simulink model "funkcija"  (R2015a)
settings: Solver=ode45  StartTime=0.0  StopTime=100.0  RelTol=1e-3
values from neighbouring files (symbols this model uses):
  teta1 = 0.5    [Parametri.m]
  teta2 = -0    (= 0)    [Parametri.m]
  v1 = 0    [Parametri.m]
  v2 = 0    [Parametri.m]
undefined symbols (not defined in the file or in its folder): A1, A2, A3, A4, l1, l2
settings Model: Creator=BLAGI  LastModifiedBy=BLAGI

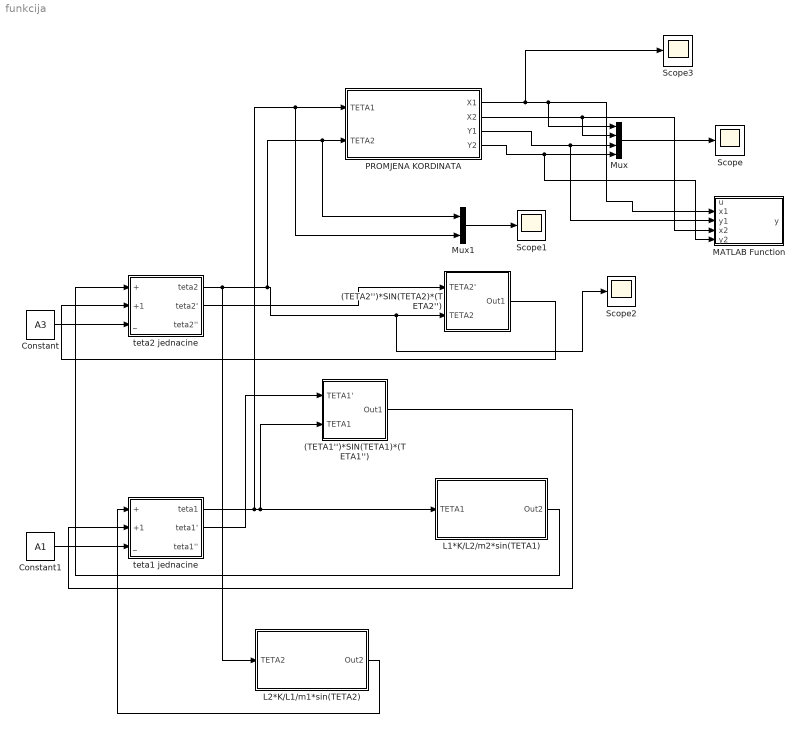
== system funkcija ==
  (TETA1'')*SIN(TETA1)*(TETA1'') : Subsystem
  (TETA2'')*SIN(TETA2)*(TETA2'') : Subsystem
  Constant : Constant  Value=A3
  Constant1 : Constant  Value=A1
  L1*K/L2/m2*sin(TETA1) : Subsystem
  L2*K/L1/m1*sin(TETA2) : Subsystem
  MATLAB Function : MATLAB Function  TreatAsAtomicUnit=on
  Mux : Mux
  Mux1 : Mux  Inputs=2
  "PROMJENA KORDINATA " : Subsystem
  Scope{,1..3} (4 alike) : Scope
      Scope settings: YMin=0  YMax=1
      Scope1 settings: YMin=0  YMax=1
      Scope2 settings: YMin=0  YMax=1  SaveName=ScopeData2
      Scope3 settings: YMin=0  YMax=1  SaveName=ScopeData3
  teta1 jednacine : Subsystem
  teta2 jednacine : Subsystem
  wires:
  Constant/1 -> teta2 jednacine/3(_)
  Constant1/1 -> teta1 jednacine/3(_)
  teta2 jednacine/1(teta2) -> L2*K/L1/m1*sin(TETA2)/1(TETA2), Mux1/1, "PROMJENA KORDINATA "/2(TETA2), Scope2/1, (TETA2'')*SIN(TETA2)*(TETA2'')/2(TETA2)
  (TETA2'')*SIN(TETA2)*(TETA2'')/1(Out1) -> teta2 jednacine/2(+1)
  L1*K/L2/m2*sin(TETA1)/1(Out2) -> teta2 jednacine/1(+)
  teta1 jednacine/2(teta1') -> (TETA1'')*SIN(TETA1)*(TETA1'')/1(TETA1')
  (TETA1'')*SIN(TETA1)*(TETA1'')/1(Out1) -> teta1 jednacine/2(+1)
  teta2 jednacine/2(teta2') -> (TETA2'')*SIN(TETA2)*(TETA2'')/1(TETA2')
  L2*K/L1/m1*sin(TETA2)/1(Out2) -> teta1 jednacine/1(+)
  Mux/1 -> Scope/1
  teta1 jednacine/1(teta1) -> Mux1/2, "PROMJENA KORDINATA "/1(TETA1), (TETA1'')*SIN(TETA1)*(TETA1'')/2(TETA1), L1*K/L2/m2*sin(TETA1)/1(TETA1)
  "PROMJENA KORDINATA "/2(X2) -> MATLAB Function/4(x2), Mux/2
  "PROMJENA KORDINATA "/3(Y1) -> MATLAB Function/3(y1), Mux/3
  "PROMJENA KORDINATA "/4(Y2) -> MATLAB Function/5(y2), Mux/4
  Mux1/1 -> Scope1/1
  "PROMJENA KORDINATA "/1(X1) -> Scope3/1, MATLAB Function/2(x1), Mux/1

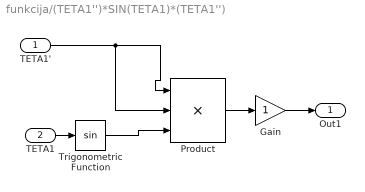
== system funkcija/(TETA1'')*SIN(TETA1)*(TETA1'') ==
  TETA1' : Inport
  TETA1 : Inport  Port=2
  Gain : Gain
  Product : Product  Inputs=3
  Trigonometric Function : Trigonometry
  Out1 : Outport
  wires:
  TETA1/1 -> Trigonometric Function/1
  Product/1 -> Gain/1
  TETA1'/1 -> Product/2, Product/1
  Trigonometric Function/1 -> Product/3
  Gain/1 -> Out1/1

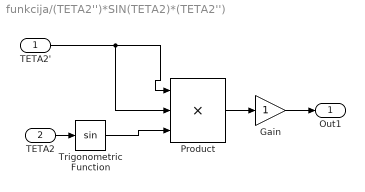
== system funkcija/(TETA2'')*SIN(TETA2)*(TETA2'') ==
  TETA2' : Inport
  TETA2 : Inport  Port=2
  Gain : Gain
  Product : Product  Inputs=3
  Trigonometric Function : Trigonometry
  Out1 : Outport
  wires:
  TETA2/1 -> Trigonometric Function/1
  Product/1 -> Gain/1
  TETA2'/1 -> Product/2, Product/1
  Trigonometric Function/1 -> Product/3
  Gain/1 -> Out1/1

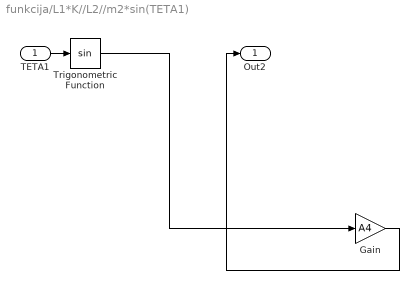
== system funkcija/L1*K//L2//m2*sin(TETA1) ==
  TETA1 : Inport
  Gain : Gain  Gain=A4
  Trigonometric Function : Trigonometry
  Out2 : Outport
  wires:
  TETA1/1 -> Trigonometric Function/1
  Trigonometric Function/1 -> Gain/1
  Gain/1 -> Out2/1

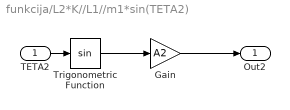
== system funkcija/L2*K//L1//m1*sin(TETA2) ==
  TETA2 : Inport
  Gain : Gain  Gain=A2
  Trigonometric Function : Trigonometry
  Out2 : Outport
  wires:
  TETA2/1 -> Trigonometric Function/1
  Trigonometric Function/1 -> Gain/1
  Gain/1 -> Out2/1

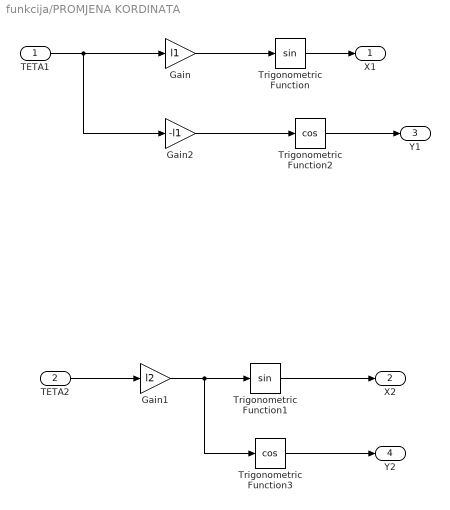
== system funkcija/PROMJENA KORDINATA  ==
  TETA1 : Inport
  TETA2 : Inport  Port=2
  Gain : Gain  Gain=l1
  Gain1 : Gain  Gain=l2
  Gain2 : Gain  Gain=-l1
  Trigonometric Function : Trigonometry
  Trigonometric Function1 : Trigonometry
  Trigonometric Function2 : Trigonometry  Operator=cos
  Trigonometric Function3 : Trigonometry  Operator=cos
  X1 : Outport
  X2 : Outport  Port=2
  Y1 : Outport  Port=3
  Y2 : Outport  Port=4
  wires:
  Gain/1 -> Trigonometric Function/1
  Trigonometric Function/1 -> X1/1
  TETA2/1 -> Gain1/1
  Gain1/1 -> Trigonometric Function3/1, Trigonometric Function1/1
  Trigonometric Function1/1 -> X2/1
  TETA1/1 -> Gain2/1, Gain/1
  Gain2/1 -> Trigonometric Function2/1
  Trigonometric Function2/1 -> Y1/1
  Trigonometric Function3/1 -> Y2/1

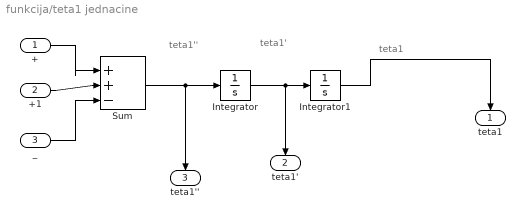
== system funkcija/teta1 jednacine ==
  note: teta1
  note: teta1'
  note: teta1''
  + : Inport
  +1 : Inport  Port=2
  _ : Inport  Port=3
  Integrator : Integrator  InitialCondition=v1
  Integrator1 : Integrator  InitialCondition=teta1  LimitOutput=on  UpperSaturationLimit=180  LowerSaturationLimit=-180
  Sum : Sum  Inputs=|++-
  teta1 : Outport
  teta1' : Outport  Port=2
  teta1'' : Outport  Port=3
  wires:
  Integrator/1 -> teta1'/1, Integrator1/1
  Sum/1 -> teta1''/1, Integrator/1
  Integrator1/1 -> teta1/1
  _/1 -> Sum/3
  +/1 -> Sum/1
  +1/1 -> Sum/2

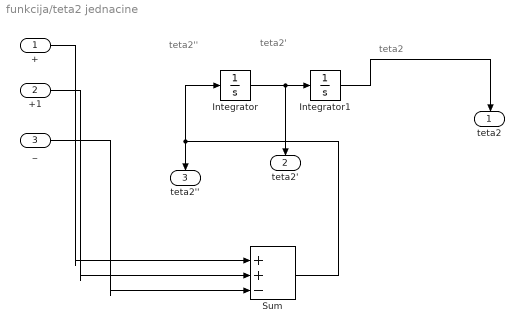
== system funkcija/teta2 jednacine ==
  note: teta2
  note: teta2'
  note: teta2''
  + : Inport
  +1 : Inport  Port=2
  _ : Inport  Port=3
  Integrator : Integrator  InitialCondition=v2  UpperSaturationLimit=360  LowerSaturationLimit=0
  Integrator1 : Integrator  InitialCondition=teta2  LimitOutput=on  UpperSaturationLimit=180  LowerSaturationLimit=-180
  Sum : Sum  Inputs=|++-
  teta2 : Outport
  teta2' : Outport  Port=2
  teta2'' : Outport  Port=3
  wires:
  Integrator/1 -> teta2'/1, Integrator1/1
  Sum/1 -> Integrator/1, teta2''/1
  Integrator1/1 -> teta2/1
  _/1 -> Sum/3
  +/1 -> Sum/1
  +1/1 -> Sum/2

== matlab function funkcija/MATLAB Function ==
  data: u input; y output; x1 input; y1 input; x2 input; y2 input
function y = fcn(u,x1,y1,x2,y2)
%#codegen
plot(x1,y1,'O');
hold
plot(x2,y2,'X');
hold

y = u;
